simulink model "dt_toy_model_simulation"  (R2024a)
settings: Solver=FixedStepAuto  StartTime=0.0  StopTime=Tsim  FixedStep=dT  RelTol=1e-3
values from neighbouring files (symbols this model uses):
  Ac = full(sysA)    [CT_and_DT_Controller.m]
  Ad = dt_ol_sys.A    [CT_and_DT_Controller.m]
  Bc = full(sysB)    [CT_and_DT_Controller.m]
  Bd = dt_ol_sys.B    [CT_and_DT_Controller.m]
  dt_Phiu1 = full(dt_Phiu{1})    [CT_and_DT_Controller.m]
  dt_Phiu2 = full(dt_Phiu{2})    [CT_and_DT_Controller.m]
  dt_Phiu3 = full(dt_Phiu{3})    [CT_and_DT_Controller.m]
  dt_Phiu4 = full(dt_Phiu{4})    [CT_and_DT_Controller.m]
  dt_Phiu5 = full(dt_Phiu{5})    [CT_and_DT_Controller.m]
  dt_Phiu6 = full(dt_Phiu{6})    [CT_and_DT_Controller.m]
  dt_Phiu7 = full(dt_Phiu{7})    [CT_and_DT_Controller.m]
  dt_Phix2 = full(dt_Phix{2})    [CT_and_DT_Controller.m]
  dt_Phix3 = full(dt_Phix{3})    [CT_and_DT_Controller.m]
  dt_Phix4 = full(dt_Phix{4})    [CT_and_DT_Controller.m]
  dt_Phix5 = full(dt_Phix{5})    [CT_and_DT_Controller.m]
  dt_Phix6 = full(dt_Phix{6})    [CT_and_DT_Controller.m]
  dt_Phix7 = full(dt_Phix{7})    [CT_and_DT_Controller.m]
  Ts = 0.2    [CT_and_DT_Controller.m]
  x0 = zeros(n,1)    [CT_and_DT_Controller.m]
(part 1 of 2)
settings Model: Creator=ralph zhao  LastModifiedBy=ralph zhao

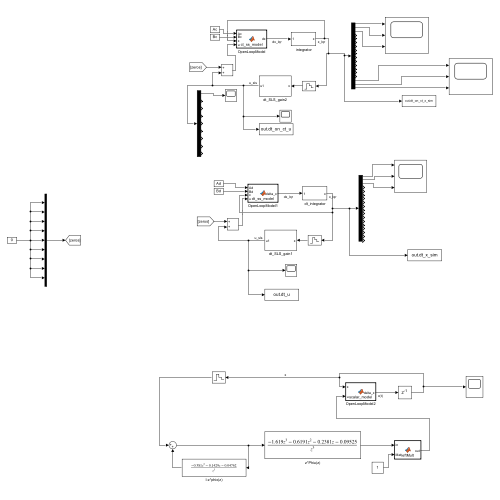
[thumbnail: Simulink's stored preview of the top-level diagram]
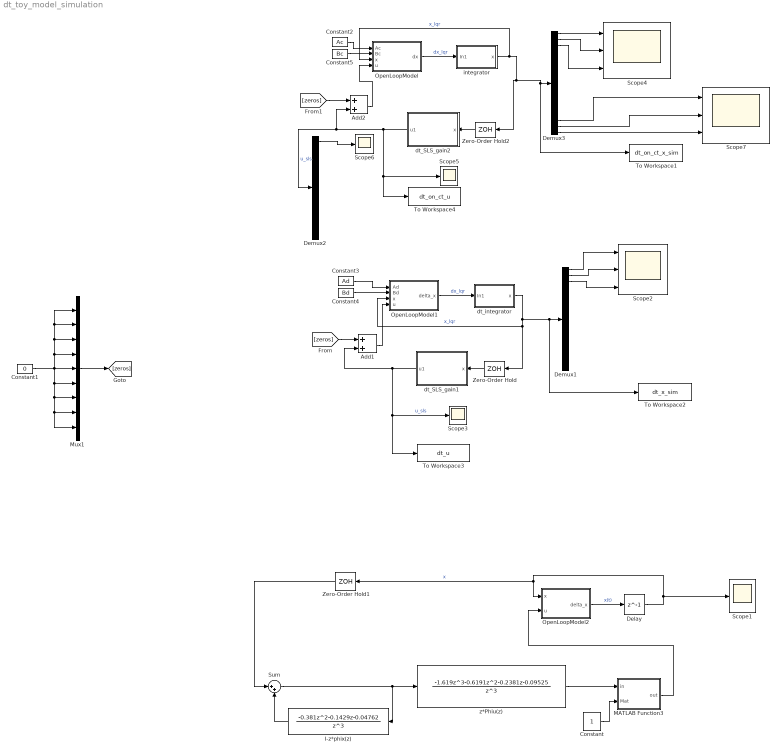
== system dt_toy_model_simulation ==
  " dt_integrator" : Subsystem
  " integrator" : Subsystem
  Add1 : Sum
  Add2 : Sum
  Constant : Constant
  Constant1 : Constant  Value=0
  Constant2 : Constant  Value=Ac
  Constant3 : Constant  Value=Ad
  Constant4 : Constant  Value=Bd
  Constant5 : Constant  Value=Bc
  Delay : Delay  DelayLength=1  InitialCondition=0.5
  Demux1 : Demux  Outputs=18
  Demux2 : Demux  Outputs=9
  Demux3 : Demux  Outputs=18
  I-z*phix(z) : DiscreteTransferFcn  Numerator=[-0.381 -0.1429 -0.04762]  Denominator=[1 0 0 0]
  MATLAB Function3 : MATLAB Function  TreatAsAtomicUnit=on
  Mux1 : Mux  Inputs=9
  OpenLoopModel : MATLAB Function  TreatAsAtomicUnit=on
  OpenLoopModel1 : MATLAB Function  TreatAsAtomicUnit=on
  OpenLoopModel2 : MATLAB Function  TreatAsAtomicUnit=on
  Scope{1,3,5..6} (4 alike) : Scope
  Scope2 : Scope  NumInputPorts=3
  Scope4 : Scope  NumInputPorts=3
  Scope7 : Scope  NumInputPorts=3
  Sum : Sum  Inputs=|++
  To Workspace1 : ToWorkspace  VariableName=dt_on_ct_x_sim  SaveFormat=Timeseries  SampleTime=-1
  To Workspace2 : ToWorkspace  VariableName=dt_x_sim  SaveFormat=Timeseries  SampleTime=-1
  To Workspace3 : ToWorkspace  VariableName=dt_u  SaveFormat=Timeseries  SampleTime=-1
  To Workspace4 : ToWorkspace  VariableName=dt_on_ct_u  SaveFormat=Timeseries  SampleTime=-1
  Zero-Order Hold : ZeroOrderHold  SampleTime=Ts
  Zero-Order Hold1 : ZeroOrderHold  SampleTime=Ts
  Zero-Order Hold2 : ZeroOrderHold  SampleTime=Ts
  dt_SLS_gain1 : Subsystem
  dt_SLS_gain2 : Subsystem
  z*Phiu(z) : DiscreteTransferFcn  Numerator=[-1.619 -0.6191 -0.2381 -0.09525]  Denominator=[1 0 0 0]
  wires:
  dt_SLS_gain1/1(u1) -> Add1/2, Scope3/1, To Workspace3/1  "u_sls"
  Add1/1 -> OpenLoopModel1/4(u)
  " dt_integrator"/1(x) -> OpenLoopModel1/3(x), Zero-Order Hold/1, Demux1/1, To Workspace2/1  "x_lqr"
  Mux1/1 -> [zeros]
  Demux1/3 -> Scope2/3
  Demux1/2 -> Scope2/2
  Demux1/1 -> Scope2/1
  OpenLoopModel1/1(delta_x) -> " dt_integrator"/1(In1)  "dx_lqr"
  Zero-Order Hold/1 -> dt_SLS_gain1/1(x)
  OpenLoopModel2/1(delta_x) -> Delay/1  "x(t)"
  Delay/1 -> Zero-Order Hold1/1, OpenLoopModel2/1(x), Scope1/1  "x"
  I-z*phix(z)/1 -> Sum/2
  Sum/1 -> I-z*phix(z)/1, z*Phiu(z)/1
  z*Phiu(z)/1 -> MATLAB Function3/1(in)
  Constant/1 -> MATLAB Function3/2(Mat)
  MATLAB Function3/1(out) -> OpenLoopModel2/2(u)
  Zero-Order Hold1/1 -> Sum/1
  Zero-Order Hold2/1 -> dt_SLS_gain2/1(x)
  OpenLoopModel/1(dx) -> " integrator"/1(In1)  "dx_lqr"
  " integrator"/1(x) -> OpenLoopModel/3(x), Zero-Order Hold2/1, To Workspace1/1, Demux3/1  "x_lqr"
  Add2/1 -> OpenLoopModel/4(u)
  dt_SLS_gain2/1(u1) -> To Workspace4/1, Scope5/1, Demux2/1, Add2/2  "u_sls"
  Constant3/1 -> OpenLoopModel1/1(Ad)
  Constant4/1 -> OpenLoopModel1/2(Bd)
  Constant1/1 -> Mux1/1, Mux1/2, Mux1/3, Mux1/4, Mux1/5, Mux1/6, Mux1/8, Mux1/9, Mux1/7
  [zeros] -> Add1/1
  [zeros] -> Add2/1
  Constant2/1 -> OpenLoopModel/1(Ac)
  Constant5/1 -> OpenLoopModel/2(Bc)
  Demux3/1 -> Scope4/1
  Demux3/2 -> Scope4/2
  Demux3/3 -> Scope4/3
  Demux2/1 -> Scope6/1
  Demux3/18 -> Scope7/3
  Demux3/17 -> Scope7/2
  Demux3/16 -> Scope7/1

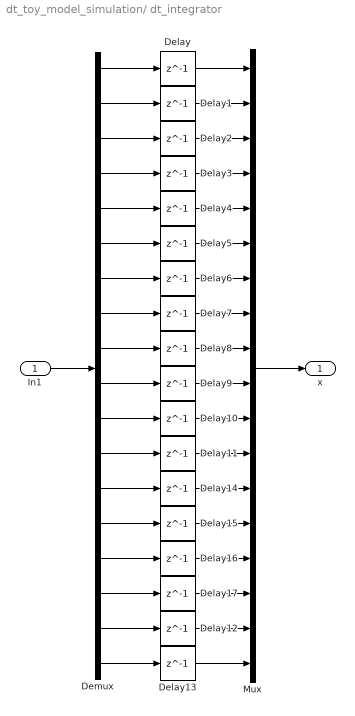
== system dt_toy_model_simulation/ dt_integrator ==
  In1 : Inport
  Delay : Delay  DelayLength=1  InitialCondition=x0(1)
  Delay1 : Delay  DelayLength=1  InitialCondition=x0(2)
  Delay10 : Delay  DelayLength=1  InitialCondition=x0(11)
  Delay11 : Delay  DelayLength=1  InitialCondition=x0(12)
  Delay12 : Delay  DelayLength=1  InitialCondition=x0(17)
  Delay13 : Delay  DelayLength=1  InitialCondition=x0(18)
  Delay14 : Delay  DelayLength=1  InitialCondition=x0(13)
  Delay15 : Delay  DelayLength=1  InitialCondition=x0(14)
  Delay16 : Delay  DelayLength=1  InitialCondition=x0(15)
  Delay17 : Delay  DelayLength=1  InitialCondition=x0(16)
  Delay2 : Delay  DelayLength=1  InitialCondition=x0(3)
  Delay3 : Delay  DelayLength=1  InitialCondition=x0(4)
  Delay4 : Delay  DelayLength=1  InitialCondition=x0(5)
  Delay5 : Delay  DelayLength=1  InitialCondition=x0(6)
  Delay6 : Delay  DelayLength=1  InitialCondition=x0(7)
  Delay7 : Delay  DelayLength=1  InitialCondition=x0(8)
  Delay8 : Delay  DelayLength=1  InitialCondition=x0(9)
  Delay9 : Delay  DelayLength=1  InitialCondition=x0(10)
  Demux : Demux  Outputs=18
  Mux : Mux  Inputs=18
  x : Outport
  wires:
  Delay2/1 -> Mux/3
  Delay1/1 -> Mux/2
  Delay/1 -> Mux/1
  Demux/3 -> Delay2/1
  In1/1 -> Demux/1
  Mux/1 -> x/1
  Demux/2 -> Delay1/1
  Demux/1 -> Delay/1
  Demux/18 -> Delay13/1
  Demux/4 -> Delay3/1
  Delay3/1 -> Mux/4
  Demux/5 -> Delay4/1
  Delay4/1 -> Mux/5
  Delay5/1 -> Mux/6
  Demux/6 -> Delay5/1
  Demux/7 -> Delay6/1
  Delay6/1 -> Mux/7
  Demux/14 -> Delay15/1
  Delay15/1 -> Mux/14
  Delay13/1 -> Mux/18
  Delay12/1 -> Mux/17
  Delay17/1 -> Mux/16
  Delay16/1 -> Mux/15
  Demux/15 -> Delay16/1
  Demux/16 -> Delay17/1
  Demux/17 -> Delay12/1
  Demux/8 -> Delay7/1
  Demux/9 -> Delay8/1
  Delay9/1 -> Mux/10
  Delay10/1 -> Mux/11
  Delay11/1 -> Mux/12
  Delay14/1 -> Mux/13
  Demux/13 -> Delay14/1
  Demux/12 -> Delay11/1
  Demux/11 -> Delay10/1
  Demux/10 -> Delay9/1
  Delay8/1 -> Mux/9
  Delay7/1 -> Mux/8

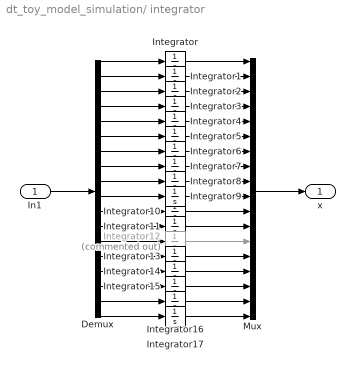
== system dt_toy_model_simulation/ integrator ==
  In1 : Inport
  Demux : Demux  Outputs=18
  Integrator : Integrator  InitialCondition=x0(1)
  Integrator1 : Integrator  InitialCondition=x0(2)
  Integrator10 : Integrator  InitialCondition=x0(11)
  Integrator11 : Integrator  InitialCondition=x0(12)
  Integrator12 : Integrator  Commented=on  InitialCondition=x0(13)
  Integrator13 : Integrator  InitialCondition=x0(14)
  Integrator14 : Integrator  InitialCondition=x0(15)
  Integrator15 : Integrator  InitialCondition=x0(16)
  Integrator16 : Integrator  InitialCondition=x0(17)
  Integrator17 : Integrator  InitialCondition=x0(18)
  Integrator2 : Integrator  InitialCondition=x0(3)
  Integrator3 : Integrator  InitialCondition=x0(4)
  Integrator4 : Integrator  InitialCondition=x0(5)
  Integrator5 : Integrator  InitialCondition=x0(6)
  Integrator6 : Integrator  InitialCondition=x0(7)
  Integrator7 : Integrator  InitialCondition=x0(8)
  Integrator8 : Integrator  InitialCondition=x0(9)
  Integrator9 : Integrator  InitialCondition=x0(10)
  Mux : Mux  Inputs=18
  x : Outport
  wires:
  Integrator2/1 -> Mux/3
  Integrator1/1 -> Mux/2
  Integrator/1 -> Mux/1
  Demux/3 -> Integrator2/1
  In1/1 -> Demux/1
  Mux/1 -> x/1
  Demux/2 -> Integrator1/1
  Demux/1 -> Integrator/1
  Demux/4 -> Integrator3/1
  Integrator3/1 -> Mux/4
  Demux/9 -> Integrator8/1
  Integrator8/1 -> Mux/9
  Demux/8 -> Integrator7/1
  Demux/7 -> Integrator6/1
  Demux/6 -> Integrator5/1
  Demux/5 -> Integrator4/1
  Integrator4/1 -> Mux/5
  Integrator5/1 -> Mux/6
  Integrator6/1 -> Mux/7
  Integrator7/1 -> Mux/8
  Demux/10 -> Integrator9/1
  Demux/11 -> Integrator10/1
  Demux/12 -> Integrator11/1
  Demux/13 -> Integrator12/1
  Demux/14 -> Integrator13/1
  Demux/15 -> Integrator14/1
  Demux/16 -> Integrator15/1
  Demux/17 -> Integrator16/1
  Demux/18 -> Integrator17/1
  Integrator17/1 -> Mux/18
  Integrator16/1 -> Mux/17
  Integrator15/1 -> Mux/16
  Integrator14/1 -> Mux/15
  Integrator13/1 -> Mux/14
  Integrator12/1 -> Mux/13
  Integrator11/1 -> Mux/12
  Integrator10/1 -> Mux/11
  Integrator9/1 -> Mux/10

== system dt_toy_model_simulation/dt_SLS_gain1 ==
  x : Inport
  Subtract1 : Sum  Inputs=+-
  z*Phi_u(z) : Subsystem
  z*Phi_x(z)-I : Subsystem
  u1 : Outport
  wires:
  z*Phi_u(z)/1(z*phi_u(z)) -> u1/1
  z*Phi_x(z)-I/1((z*phi_x(z)-I)) -> Subtract1/2
  Subtract1/1 -> z*Phi_x(z)-I/1(v), z*Phi_u(z)/1(I)  "v"
  x/1 -> Subtract1/1

== system dt_toy_model_simulation/dt_SLS_gain2 ==
  x : Inport
  Subtract1 : Sum  Inputs=+-
  z*Phi_u(z) : Subsystem
  z*Phi_x(z)-I : Subsystem
  u1 : Outport
  wires:
  x/1 -> Subtract1/1
  Subtract1/1 -> z*Phi_u(z)/1(I), z*Phi_x(z)-I/1(v)  "v"
  z*Phi_x(z)-I/1((z*phi_x(z)-I)) -> Subtract1/2
  z*Phi_u(z)/1(z*phi_u(z)) -> u1/1

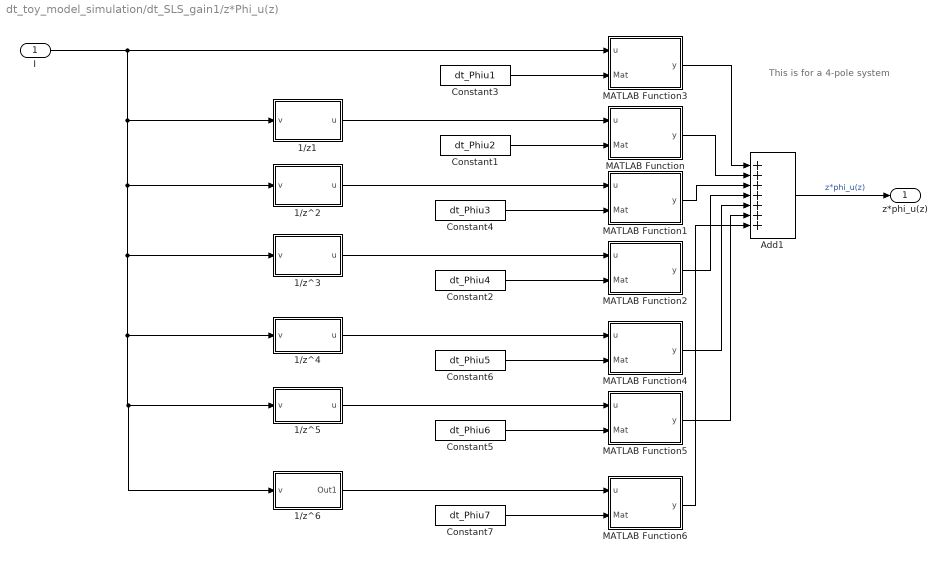
== system dt_toy_model_simulation/dt_SLS_gain1/z*Phi_u(z) ==
  note: This is for a 4-pole
      |  system
  I : Inport
  1/z1 : Subsystem
  1/z^2 : Subsystem
  1/z^3 : Subsystem
  1/z^4 : Subsystem
  1/z^5 : Subsystem
  1/z^6 : Subsystem
  Add1 : Sum  Inputs=+++++++
  Constant1 : Constant  Value=dt_Phiu2
  Constant2 : Constant  Value=dt_Phiu4
  Constant3 : Constant  Value=dt_Phiu1
  Constant4 : Constant  Value=dt_Phiu3
  Constant5 : Constant  Value=dt_Phiu6
  Constant6 : Constant  Value=dt_Phiu5
  Constant7 : Constant  Value=dt_Phiu7
  MATLAB Function : MATLAB Function  TreatAsAtomicUnit=on
  MATLAB Function1 : MATLAB Function  TreatAsAtomicUnit=on
  MATLAB Function2 : MATLAB Function  TreatAsAtomicUnit=on
  MATLAB Function3 : MATLAB Function  TreatAsAtomicUnit=on
  MATLAB Function4 : MATLAB Function  TreatAsAtomicUnit=on
  MATLAB Function5 : MATLAB Function  TreatAsAtomicUnit=on
  MATLAB Function6 : MATLAB Function  TreatAsAtomicUnit=on
  z*phi_u(z) : Outport
  wires:
  Constant7/1 -> MATLAB Function6/2(Mat)
  MATLAB Function6/1(y) -> Add1/7
  1/z^6/1(Out1) -> MATLAB Function6/1(u)
  I/1 -> MATLAB Function3/1(u), 1/z^2/1(v), 1/z^3/1(v), 1/z^5/1(v), 1/z^6/1(v), 1/z^4/1(v), 1/z1/1(v)
  Constant4/1 -> MATLAB Function1/2(Mat)
  1/z^2/1(u) -> MATLAB Function1/1(u)
  Constant1/1 -> MATLAB Function/2(Mat)
  Constant2/1 -> MATLAB Function2/2(Mat)
  1/z1/1(u) -> MATLAB Function/1(u)
  Add1/1 -> z*phi_u(z)/1  "z*phi_u(z)"
  MATLAB Function2/1(y) -> Add1/4
  MATLAB Function1/1(y) -> Add1/3
  MATLAB Function/1(y) -> Add1/2
  MATLAB Function3/1(y) -> Add1/1
  Constant3/1 -> MATLAB Function3/2(Mat)
  1/z^3/1(u) -> MATLAB Function2/1(u)
  1/z^5/1(u) -> MATLAB Function5/1(u)
  MATLAB Function4/1(y) -> Add1/5
  MATLAB Function5/1(y) -> Add1/6
  Constant5/1 -> MATLAB Function5/2(Mat)
  1/z^4/1(u) -> MATLAB Function4/1(u)
  Constant6/1 -> MATLAB Function4/2(Mat)

== system dt_toy_model_simulation/dt_SLS_gain1/z*Phi_x(z)-I ==
  note: This is for a 4-pole system
  v : Inport
  1/z : Subsystem
  1/z^2 : Subsystem
  1/z^3 : Subsystem
  1/z^4 : Subsystem
  1/z^5 : Subsystem
  1/z^6 : Subsystem
  Add1 : Sum  Inputs=++++++
  Constant1 : Constant  Value=dt_Phix2
  Constant2 : Constant  Value=dt_Phix4
  Constant3 : Constant  Value=dt_Phix7
  Constant4 : Constant  Value=dt_Phix3
  Constant5 : Constant  Value=dt_Phix6
  Constant6 : Constant  Value=dt_Phix5
  MATLAB Function : MATLAB Function  TreatAsAtomicUnit=on
  MATLAB Function1 : MATLAB Function  TreatAsAtomicUnit=on
  MATLAB Function2 : MATLAB Function  TreatAsAtomicUnit=on
  MATLAB Function3 : MATLAB Function  TreatAsAtomicUnit=on
  MATLAB Function4 : MATLAB Function  TreatAsAtomicUnit=on
  MATLAB Function5 : MATLAB Function  TreatAsAtomicUnit=on
  (z*phi_x(z)-I) : Outport
  wires:
  MATLAB Function3/1(y) -> Add1/6
  v/1 -> 1/z^5/1(v), 1/z^6/1(v), 1/z^4/1(v), 1/z^3/1(v), 1/z^2/1(v), 1/z/1(v)
  1/z^6/1(Out1) -> MATLAB Function3/1(u)
  Constant3/1 -> MATLAB Function3/2(Mat)
  1/z^2/1(Out1) -> MATLAB Function1/1(u)
  Add1/1 -> (z*phi_x(z)-I)/1
  Constant1/1 -> MATLAB Function/2(Mat)
  1/z/1(Out1) -> MATLAB Function/1(u)
  MATLAB Function/1(y) -> Add1/1
  Constant4/1 -> MATLAB Function1/2(Mat)
  MATLAB Function1/1(y) -> Add1/2
  1/z^3/1(Out1) -> MATLAB Function2/1(u)
  Constant2/1 -> MATLAB Function2/2(Mat)
  MATLAB Function2/1(y) -> Add1/3
  Constant5/1 -> MATLAB Function5/2(Mat)
  1/z^5/1(Out1) -> MATLAB Function5/1(u)
  Constant6/1 -> MATLAB Function4/2(Mat)
  1/z^4/1(Out1) -> MATLAB Function4/1(u)
  MATLAB Function4/1(y) -> Add1/4
  MATLAB Function5/1(y) -> Add1/5

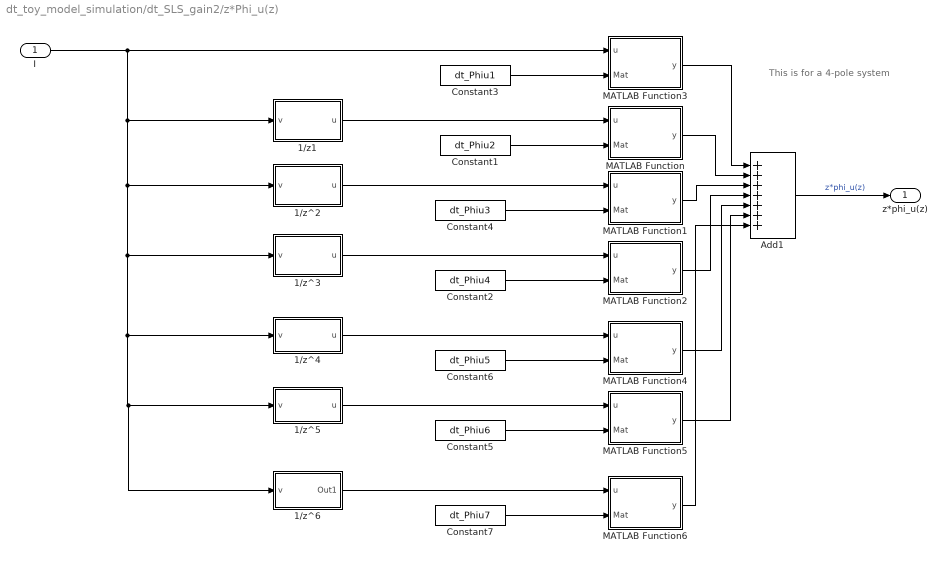
== system dt_toy_model_simulation/dt_SLS_gain2/z*Phi_u(z) ==
  note: This is for a 4-pole
      |  system
  I : Inport
  1/z1 : Subsystem
  1/z^2 : Subsystem
  1/z^3 : Subsystem
  1/z^4 : Subsystem
  1/z^5 : Subsystem
  1/z^6 : Subsystem
  Add1 : Sum  Inputs=+++++++
  Constant1 : Constant  Value=dt_Phiu2
  Constant2 : Constant  Value=dt_Phiu4
  Constant3 : Constant  Value=dt_Phiu1
  Constant4 : Constant  Value=dt_Phiu3
  Constant5 : Constant  Value=dt_Phiu6
  Constant6 : Constant  Value=dt_Phiu5
  Constant7 : Constant  Value=dt_Phiu7
  MATLAB Function : MATLAB Function  TreatAsAtomicUnit=on
  MATLAB Function1 : MATLAB Function  TreatAsAtomicUnit=on
  MATLAB Function2 : MATLAB Function  TreatAsAtomicUnit=on
  MATLAB Function3 : MATLAB Function  TreatAsAtomicUnit=on
  MATLAB Function4 : MATLAB Function  TreatAsAtomicUnit=on
  MATLAB Function5 : MATLAB Function  TreatAsAtomicUnit=on
  MATLAB Function6 : MATLAB Function  TreatAsAtomicUnit=on
  z*phi_u(z) : Outport
  wires:
  Constant6/1 -> MATLAB Function4/2(Mat)
  1/z^4/1(u) -> MATLAB Function4/1(u)
  Constant5/1 -> MATLAB Function5/2(Mat)
  MATLAB Function5/1(y) -> Add1/6
  MATLAB Function4/1(y) -> Add1/5
  1/z^5/1(u) -> MATLAB Function5/1(u)
  1/z^3/1(u) -> MATLAB Function2/1(u)
  Constant3/1 -> MATLAB Function3/2(Mat)
  MATLAB Function3/1(y) -> Add1/1
  MATLAB Function/1(y) -> Add1/2
  MATLAB Function1/1(y) -> Add1/3
  MATLAB Function2/1(y) -> Add1/4
  Add1/1 -> z*phi_u(z)/1  "z*phi_u(z)"
  1/z1/1(u) -> MATLAB Function/1(u)
  Constant2/1 -> MATLAB Function2/2(Mat)
  Constant1/1 -> MATLAB Function/2(Mat)
  1/z^2/1(u) -> MATLAB Function1/1(u)
  Constant4/1 -> MATLAB Function1/2(Mat)
  I/1 -> 1/z1/1(v), 1/z^4/1(v), 1/z^6/1(v), 1/z^5/1(v), 1/z^3/1(v), 1/z^2/1(v), MATLAB Function3/1(u)
  1/z^6/1(Out1) -> MATLAB Function6/1(u)
  MATLAB Function6/1(y) -> Add1/7
  Constant7/1 -> MATLAB Function6/2(Mat)

== system dt_toy_model_simulation/dt_SLS_gain2/z*Phi_x(z)-I ==
  note: This is for a 4-pole system
  v : Inport
  1/z : Subsystem
  1/z^2 : Subsystem
  1/z^3 : Subsystem
  1/z^4 : Subsystem
  1/z^5 : Subsystem
  1/z^6 : Subsystem
  Add1 : Sum  Inputs=++++++
  Constant1 : Constant  Value=dt_Phix2
  Constant2 : Constant  Value=dt_Phix4
  Constant3 : Constant  Value=dt_Phix7
  Constant4 : Constant  Value=dt_Phix3
  Constant5 : Constant  Value=dt_Phix6
  Constant6 : Constant  Value=dt_Phix5
  MATLAB Function : MATLAB Function  TreatAsAtomicUnit=on
  MATLAB Function1 : MATLAB Function  TreatAsAtomicUnit=on
  MATLAB Function2 : MATLAB Function  TreatAsAtomicUnit=on
  MATLAB Function3 : MATLAB Function  TreatAsAtomicUnit=on
  MATLAB Function4 : MATLAB Function  TreatAsAtomicUnit=on
  MATLAB Function5 : MATLAB Function  TreatAsAtomicUnit=on
  (z*phi_x(z)-I) : Outport
  wires:
  MATLAB Function5/1(y) -> Add1/5
  MATLAB Function4/1(y) -> Add1/4
  1/z^4/1(Out1) -> MATLAB Function4/1(u)
  Constant6/1 -> MATLAB Function4/2(Mat)
  1/z^5/1(Out1) -> MATLAB Function5/1(u)
  Constant5/1 -> MATLAB Function5/2(Mat)
  MATLAB Function2/1(y) -> Add1/3
  Constant2/1 -> MATLAB Function2/2(Mat)
  1/z^3/1(Out1) -> MATLAB Function2/1(u)
  MATLAB Function1/1(y) -> Add1/2
  Constant4/1 -> MATLAB Function1/2(Mat)
  MATLAB Function/1(y) -> Add1/1
  1/z/1(Out1) -> MATLAB Function/1(u)
  Constant1/1 -> MATLAB Function/2(Mat)
  Add1/1 -> (z*phi_x(z)-I)/1
  1/z^2/1(Out1) -> MATLAB Function1/1(u)
  Constant3/1 -> MATLAB Function3/2(Mat)
  1/z^6/1(Out1) -> MATLAB Function3/1(u)
  v/1 -> 1/z/1(v), 1/z^2/1(v), 1/z^3/1(v), 1/z^4/1(v), 1/z^6/1(v), 1/z^5/1(v)
  MATLAB Function3/1(y) -> Add1/6

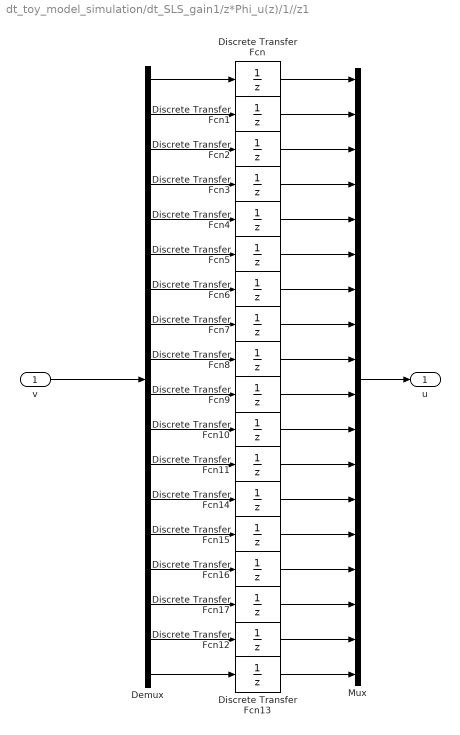
== system dt_toy_model_simulation/dt_SLS_gain1/z*Phi_u(z)/1//z1 ==
  v : Inport
  Demux : Demux  Outputs=18
  Discrete Transfer Fcn{,1..17} (18 alike) : DiscreteTransferFcn  Denominator=[1 0]
  Mux : Mux  Inputs=18
  u : Outport
  wires:
  Discrete Transfer Fcn1/1 -> Mux/2
  Demux/1 -> Discrete Transfer Fcn/1
  Discrete Transfer Fcn2/1 -> Mux/3
  Discrete Transfer Fcn/1 -> Mux/1
  Demux/2 -> Discrete Transfer Fcn1/1
  Demux/3 -> Discrete Transfer Fcn2/1
  Mux/1 -> u/1
  v/1 -> Demux/1
  Demux/4 -> Discrete Transfer Fcn3/1
  Demux/5 -> Discrete Transfer Fcn4/1
  Demux/6 -> Discrete Transfer Fcn5/1
  Demux/7 -> Discrete Transfer Fcn6/1
  Demux/8 -> Discrete Transfer Fcn7/1
  Demux/9 -> Discrete Transfer Fcn8/1
  Demux/10 -> Discrete Transfer Fcn9/1
  Demux/11 -> Discrete Transfer Fcn10/1
  Demux/12 -> Discrete Transfer Fcn11/1
  Demux/13 -> Discrete Transfer Fcn14/1
  Demux/14 -> Discrete Transfer Fcn15/1
  Demux/15 -> Discrete Transfer Fcn16/1
  Demux/16 -> Discrete Transfer Fcn17/1
  Demux/17 -> Discrete Transfer Fcn12/1
  Demux/18 -> Discrete Transfer Fcn13/1
  Discrete Transfer Fcn13/1 -> Mux/18
  Discrete Transfer Fcn12/1 -> Mux/17
  Discrete Transfer Fcn17/1 -> Mux/16
  Discrete Transfer Fcn16/1 -> Mux/15
  Discrete Transfer Fcn15/1 -> Mux/14
  Discrete Transfer Fcn14/1 -> Mux/13
  Discrete Transfer Fcn3/1 -> Mux/4
  Discrete Transfer Fcn4/1 -> Mux/5
  Discrete Transfer Fcn5/1 -> Mux/6
  Discrete Transfer Fcn6/1 -> Mux/7
  Discrete Transfer Fcn7/1 -> Mux/8
  Discrete Transfer Fcn8/1 -> Mux/9
  Discrete Transfer Fcn9/1 -> Mux/10
  Discrete Transfer Fcn10/1 -> Mux/11
  Discrete Transfer Fcn11/1 -> Mux/12

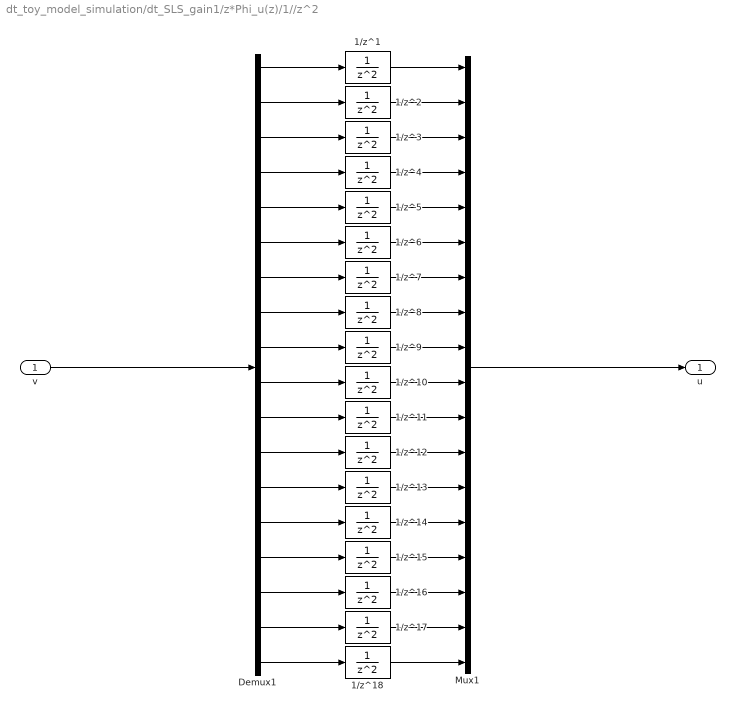
== system dt_toy_model_simulation/dt_SLS_gain1/z*Phi_u(z)/1//z^2 ==
  v : Inport
  1/z^{1..18} (18 alike) : DiscreteTransferFcn  Denominator=[1 0 0]
  Demux1 : Demux  Outputs=18
  Mux1 : Mux  Inputs=18
  u : Outport
  wires:
  Demux1/7 -> 1/z^7/1
  1/z^16/1 -> Mux1/16
  Demux1/10 -> 1/z^10/1
  1/z^17/1 -> Mux1/17
  Demux1/14 -> 1/z^14/1
  Demux1/6 -> 1/z^6/1
  1/z^13/1 -> Mux1/13
  Mux1/1 -> u/1
  Demux1/2 -> 1/z^2/1
  Demux1/1 -> 1/z^1/1
  1/z^1/1 -> Mux1/1
  1/z^6/1 -> Mux1/6
  Demux1/13 -> 1/z^13/1
  1/z^11/1 -> Mux1/11
  1/z^15/1 -> Mux1/15
  1/z^7/1 -> Mux1/7
  Demux1/12 -> 1/z^12/1
  1/z^5/1 -> Mux1/5
  Demux1/5 -> 1/z^5/1
  Demux1/9 -> 1/z^9/1
  1/z^10/1 -> Mux1/10
  Demux1/16 -> 1/z^16/1
  Demux1/4 -> 1/z^4/1
  1/z^14/1 -> Mux1/14
  1/z^2/1 -> Mux1/2
  1/z^18/1 -> Mux1/18
  v/1 -> Demux1/1
  Demux1/8 -> 1/z^8/1
  1/z^3/1 -> Mux1/3
  1/z^12/1 -> Mux1/12
  1/z^8/1 -> Mux1/8
  1/z^4/1 -> Mux1/4
  Demux1/3 -> 1/z^3/1
  Demux1/11 -> 1/z^11/1
  Demux1/18 -> 1/z^18/1
  1/z^9/1 -> Mux1/9
  Demux1/17 -> 1/z^17/1
  Demux1/15 -> 1/z^15/1

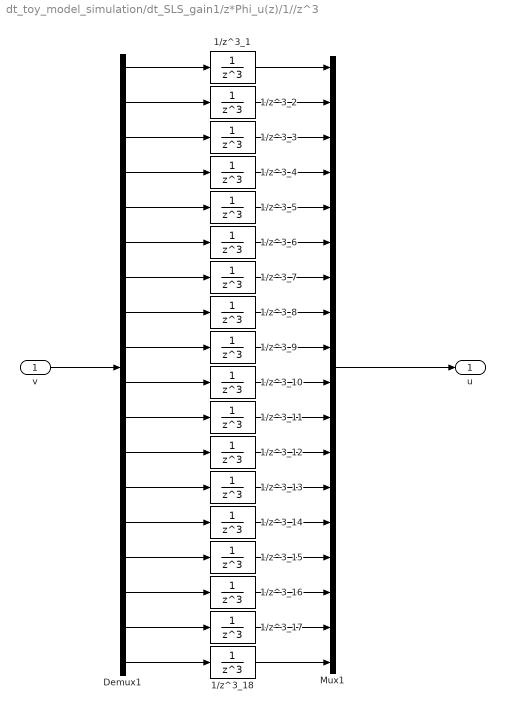
== system dt_toy_model_simulation/dt_SLS_gain1/z*Phi_u(z)/1//z^3 ==
  v : Inport
  1/z^3_{1..18} (18 alike) : DiscreteTransferFcn  Denominator=[1 0 0 0]
  Demux1 : Demux  Outputs=18
  Mux1 : Mux  Inputs=18
  u : Outport
  wires:
  Demux1/8 -> 1/z^3_8/1
  1/z^3_8/1 -> Mux1/8
  Demux1/4 -> 1/z^3_4/1
  1/z^3_5/1 -> Mux1/5
  1/z^3_18/1 -> Mux1/18
  1/z^3_17/1 -> Mux1/17
  Demux1/5 -> 1/z^3_5/1
  Demux1/17 -> 1/z^3_17/1
  Demux1/14 -> 1/z^3_14/1
  1/z^3_16/1 -> Mux1/16
  1/z^3_14/1 -> Mux1/14
  Demux1/11 -> 1/z^3_11/1
  1/z^3_11/1 -> Mux1/11
  Demux1/16 -> 1/z^3_16/1
  1/z^3_4/1 -> Mux1/4
  1/z^3_10/1 -> Mux1/10
  Demux1/18 -> 1/z^3_18/1
  Demux1/13 -> 1/z^3_13/1
  1/z^3_13/1 -> Mux1/13
  1/z^3_12/1 -> Mux1/12
  Demux1/12 -> 1/z^3_12/1
  Demux1/15 -> 1/z^3_15/1
  1/z^3_15/1 -> Mux1/15
  Mux1/1 -> u/1
  1/z^3_6/1 -> Mux1/6
  1/z^3_2/1 -> Mux1/2
  Demux1/2 -> 1/z^3_2/1
  Demux1/6 -> 1/z^3_6/1
  v/1 -> Demux1/1
  1/z^3_1/1 -> Mux1/1
  Demux1/10 -> 1/z^3_10/1
  Demux1/1 -> 1/z^3_1/1
  1/z^3_3/1 -> Mux1/3
  1/z^3_7/1 -> Mux1/7
  Demux1/7 -> 1/z^3_7/1
  Demux1/9 -> 1/z^3_9/1
  1/z^3_9/1 -> Mux1/9
  Demux1/3 -> 1/z^3_3/1

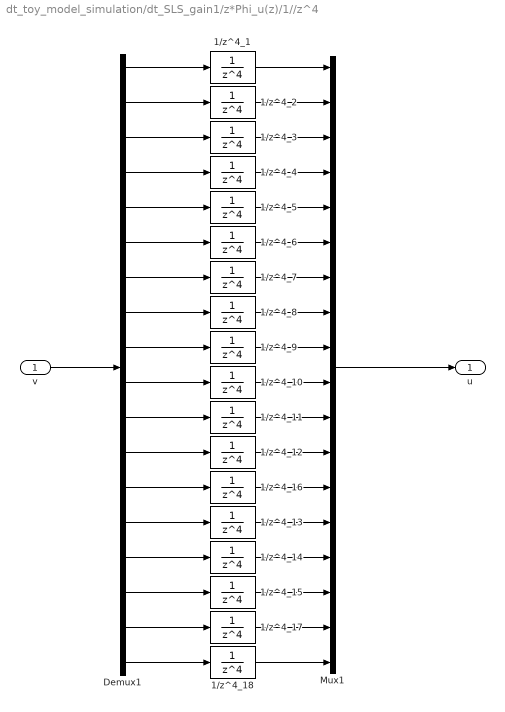
== system dt_toy_model_simulation/dt_SLS_gain1/z*Phi_u(z)/1//z^4 ==
  v : Inport
  1/z^4_{1..18} (18 alike) : DiscreteTransferFcn  Denominator=[1 0 0 0 0]
  Demux1 : Demux  Outputs=18
  Mux1 : Mux  Inputs=18
  u : Outport
  wires:
  Demux1/3 -> 1/z^4_3/1
  1/z^4_9/1 -> Mux1/9
  Demux1/9 -> 1/z^4_9/1
  Demux1/7 -> 1/z^4_7/1
  1/z^4_7/1 -> Mux1/7
  1/z^4_3/1 -> Mux1/3
  Demux1/1 -> 1/z^4_1/1
  Demux1/10 -> 1/z^4_10/1
  1/z^4_1/1 -> Mux1/1
  v/1 -> Demux1/1
  Demux1/6 -> 1/z^4_6/1
  Demux1/2 -> 1/z^4_2/1
  1/z^4_2/1 -> Mux1/2
  1/z^4_6/1 -> Mux1/6
  Mux1/1 -> u/1
  1/z^4_14/1 -> Mux1/15
  Demux1/15 -> 1/z^4_14/1
  Demux1/12 -> 1/z^4_12/1
  1/z^4_12/1 -> Mux1/12
  1/z^4_16/1 -> Mux1/13
  Demux1/13 -> 1/z^4_16/1
  Demux1/18 -> 1/z^4_18/1
  1/z^4_10/1 -> Mux1/10
  1/z^4_4/1 -> Mux1/4
  Demux1/16 -> 1/z^4_15/1
  1/z^4_11/1 -> Mux1/11
  Demux1/11 -> 1/z^4_11/1
  1/z^4_13/1 -> Mux1/14
  1/z^4_15/1 -> Mux1/16
  Demux1/14 -> 1/z^4_13/1
  Demux1/17 -> 1/z^4_17/1
  Demux1/5 -> 1/z^4_5/1
  1/z^4_17/1 -> Mux1/17
  1/z^4_18/1 -> Mux1/18
  1/z^4_5/1 -> Mux1/5
  Demux1/4 -> 1/z^4_4/1
  1/z^4_8/1 -> Mux1/8
  Demux1/8 -> 1/z^4_8/1

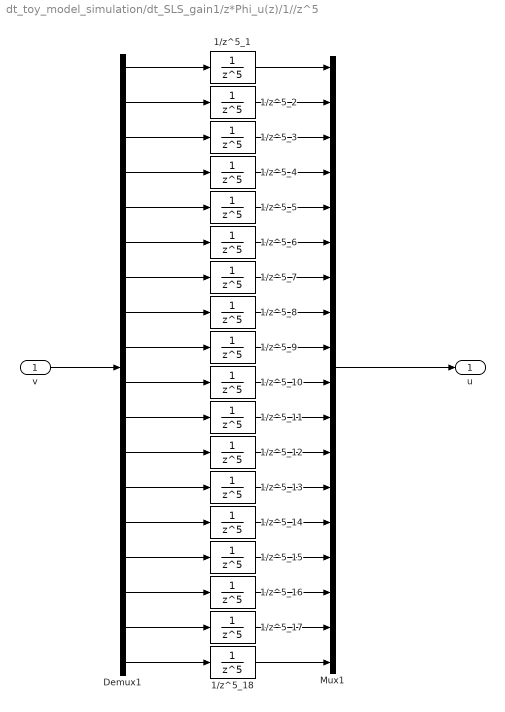
== system dt_toy_model_simulation/dt_SLS_gain1/z*Phi_u(z)/1//z^5 ==
  v : Inport
  1/z^5_{1..18} (18 alike) : DiscreteTransferFcn  Denominator=[1 0 0 0 0 0]
  Demux1 : Demux  Outputs=18
  Mux1 : Mux  Inputs=18
  u : Outport
  wires:
  Demux1/8 -> 1/z^5_8/1
  1/z^5_8/1 -> Mux1/8
  Demux1/4 -> 1/z^5_4/1
  1/z^5_5/1 -> Mux1/5
  1/z^5_18/1 -> Mux1/18
  1/z^5_17/1 -> Mux1/17
  Demux1/5 -> 1/z^5_5/1
  Demux1/17 -> 1/z^5_17/1
  Demux1/14 -> 1/z^5_14/1
  1/z^5_16/1 -> Mux1/16
  1/z^5_14/1 -> Mux1/14
  Demux1/11 -> 1/z^5_11/1
  1/z^5_11/1 -> Mux1/11
  Demux1/16 -> 1/z^5_16/1
  1/z^5_4/1 -> Mux1/4
  1/z^5_10/1 -> Mux1/10
  Demux1/18 -> 1/z^5_18/1
  Demux1/13 -> 1/z^5_13/1
  1/z^5_13/1 -> Mux1/13
  1/z^5_12/1 -> Mux1/12
  Demux1/12 -> 1/z^5_12/1
  Demux1/15 -> 1/z^5_15/1
  1/z^5_15/1 -> Mux1/15
  Mux1/1 -> u/1
  1/z^5_6/1 -> Mux1/6
  1/z^5_2/1 -> Mux1/2
  Demux1/2 -> 1/z^5_2/1
  Demux1/6 -> 1/z^5_6/1
  v/1 -> Demux1/1
  1/z^5_1/1 -> Mux1/1
  Demux1/10 -> 1/z^5_10/1
  Demux1/1 -> 1/z^5_1/1
  1/z^5_3/1 -> Mux1/3
  1/z^5_7/1 -> Mux1/7
  Demux1/7 -> 1/z^5_7/1
  Demux1/9 -> 1/z^5_9/1
  1/z^5_9/1 -> Mux1/9
  Demux1/3 -> 1/z^5_3/1

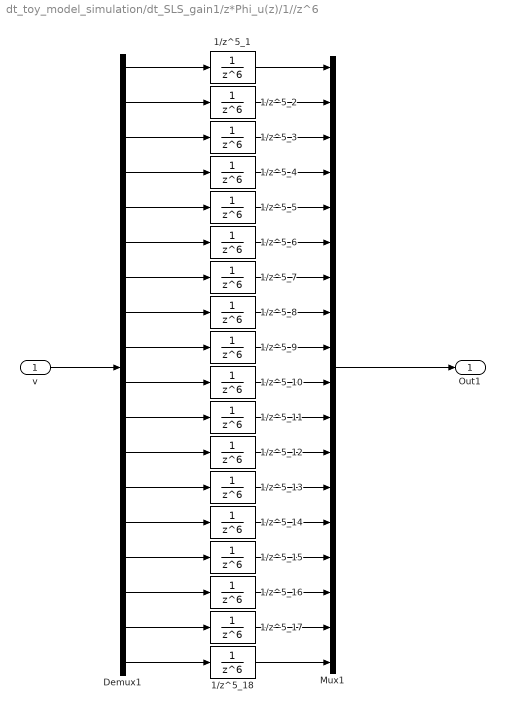
== system dt_toy_model_simulation/dt_SLS_gain1/z*Phi_u(z)/1//z^6 ==
  v : Inport
  1/z^5_{1..18} (18 alike) : DiscreteTransferFcn  Denominator=[1 0 0 0 0 0 0]
  Demux1 : Demux  Outputs=18
  Mux1 : Mux  Inputs=18
  Out1 : Outport
  wires:
  Demux1/3 -> 1/z^5_3/1
  1/z^5_9/1 -> Mux1/9
  Demux1/9 -> 1/z^5_9/1
  Demux1/7 -> 1/z^5_7/1
  1/z^5_7/1 -> Mux1/7
  1/z^5_3/1 -> Mux1/3
  Demux1/1 -> 1/z^5_1/1
  Demux1/10 -> 1/z^5_10/1
  1/z^5_1/1 -> Mux1/1
  v/1 -> Demux1/1
  Demux1/6 -> 1/z^5_6/1
  Demux1/2 -> 1/z^5_2/1
  1/z^5_2/1 -> Mux1/2
  1/z^5_6/1 -> Mux1/6
  Mux1/1 -> Out1/1
  1/z^5_15/1 -> Mux1/15
  Demux1/15 -> 1/z^5_15/1
  Demux1/12 -> 1/z^5_12/1
  1/z^5_12/1 -> Mux1/12
  1/z^5_13/1 -> Mux1/13
  Demux1/13 -> 1/z^5_13/1
  Demux1/18 -> 1/z^5_18/1
  1/z^5_10/1 -> Mux1/10
  1/z^5_4/1 -> Mux1/4
  Demux1/16 -> 1/z^5_16/1
  1/z^5_11/1 -> Mux1/11
  Demux1/11 -> 1/z^5_11/1
  1/z^5_14/1 -> Mux1/14
  1/z^5_16/1 -> Mux1/16
  Demux1/14 -> 1/z^5_14/1
  Demux1/17 -> 1/z^5_17/1
  Demux1/5 -> 1/z^5_5/1
  1/z^5_17/1 -> Mux1/17
  1/z^5_18/1 -> Mux1/18
  1/z^5_5/1 -> Mux1/5
  Demux1/4 -> 1/z^5_4/1
  1/z^5_8/1 -> Mux1/8
  Demux1/8 -> 1/z^5_8/1

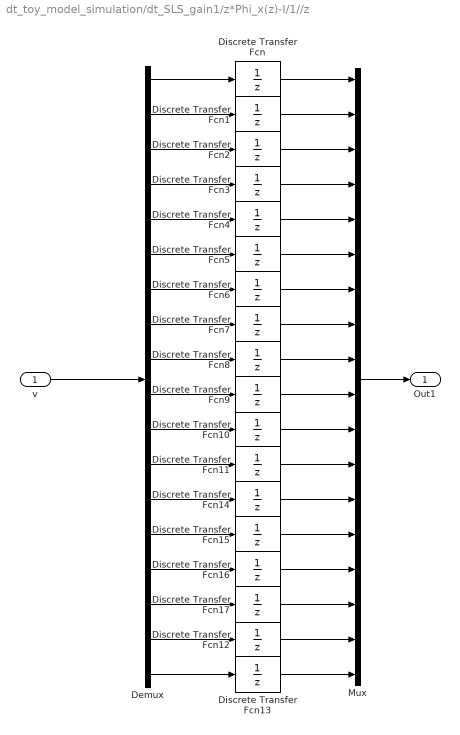
== system dt_toy_model_simulation/dt_SLS_gain1/z*Phi_x(z)-I/1//z ==
  v : Inport
  Demux : Demux  Outputs=18
  Discrete Transfer Fcn{,1..17} (18 alike) : DiscreteTransferFcn  Denominator=[1 0]
  Mux : Mux  Inputs=18
  Out1 : Outport
  wires:
  Discrete Transfer Fcn1/1 -> Mux/2
  Demux/1 -> Discrete Transfer Fcn/1
  Discrete Transfer Fcn2/1 -> Mux/3
  Discrete Transfer Fcn/1 -> Mux/1
  Demux/2 -> Discrete Transfer Fcn1/1
  Demux/3 -> Discrete Transfer Fcn2/1
  Mux/1 -> Out1/1
  v/1 -> Demux/1
  Demux/4 -> Discrete Transfer Fcn3/1
  Demux/5 -> Discrete Transfer Fcn4/1
  Demux/6 -> Discrete Transfer Fcn5/1
  Demux/7 -> Discrete Transfer Fcn6/1
  Demux/8 -> Discrete Transfer Fcn7/1
  Demux/9 -> Discrete Transfer Fcn8/1
  Demux/10 -> Discrete Transfer Fcn9/1
  Demux/11 -> Discrete Transfer Fcn10/1
  Demux/12 -> Discrete Transfer Fcn11/1
  Demux/13 -> Discrete Transfer Fcn14/1
  Demux/14 -> Discrete Transfer Fcn15/1
  Demux/15 -> Discrete Transfer Fcn16/1
  Demux/16 -> Discrete Transfer Fcn17/1
  Demux/17 -> Discrete Transfer Fcn12/1
  Demux/18 -> Discrete Transfer Fcn13/1
  Discrete Transfer Fcn13/1 -> Mux/18
  Discrete Transfer Fcn12/1 -> Mux/17
  Discrete Transfer Fcn17/1 -> Mux/16
  Discrete Transfer Fcn16/1 -> Mux/15
  Discrete Transfer Fcn15/1 -> Mux/14
  Discrete Transfer Fcn14/1 -> Mux/13
  Discrete Transfer Fcn3/1 -> Mux/4
  Discrete Transfer Fcn4/1 -> Mux/5
  Discrete Transfer Fcn5/1 -> Mux/6
  Discrete Transfer Fcn6/1 -> Mux/7
  Discrete Transfer Fcn7/1 -> Mux/8
  Discrete Transfer Fcn8/1 -> Mux/9
  Discrete Transfer Fcn9/1 -> Mux/10
  Discrete Transfer Fcn10/1 -> Mux/11
  Discrete Transfer Fcn11/1 -> Mux/12

== system dt_toy_model_simulation/dt_SLS_gain1/z*Phi_x(z)-I/1//z^2 ==
  v : Inport
  1/z^{1..18} (18 alike) : DiscreteTransferFcn  Denominator=[1 0 0]
  Demux1 : Demux  Outputs=18
  Mux1 : Mux  Inputs=18
  Out1 : Outport
  wires:
  Demux1/7 -> 1/z^7/1
  1/z^16/1 -> Mux1/16
  Demux1/10 -> 1/z^10/1
  1/z^17/1 -> Mux1/17
  Demux1/14 -> 1/z^14/1
  Demux1/6 -> 1/z^6/1
  1/z^13/1 -> Mux1/13
  Mux1/1 -> Out1/1
  Demux1/2 -> 1/z^2/1
  Demux1/1 -> 1/z^1/1
  1/z^1/1 -> Mux1/1
  1/z^6/1 -> Mux1/6
  Demux1/13 -> 1/z^13/1
  1/z^11/1 -> Mux1/11
  1/z^15/1 -> Mux1/15
  1/z^7/1 -> Mux1/7
  Demux1/12 -> 1/z^12/1
  1/z^5/1 -> Mux1/5
  Demux1/5 -> 1/z^5/1
  Demux1/9 -> 1/z^9/1
  1/z^10/1 -> Mux1/10
  Demux1/16 -> 1/z^16/1
  Demux1/4 -> 1/z^4/1
  1/z^14/1 -> Mux1/14
  1/z^2/1 -> Mux1/2
  1/z^18/1 -> Mux1/18
  v/1 -> Demux1/1
  Demux1/8 -> 1/z^8/1
  1/z^3/1 -> Mux1/3
  1/z^12/1 -> Mux1/12
  1/z^8/1 -> Mux1/8
  1/z^4/1 -> Mux1/4
  Demux1/3 -> 1/z^3/1
  Demux1/11 -> 1/z^11/1
  Demux1/18 -> 1/z^18/1
  1/z^9/1 -> Mux1/9
  Demux1/17 -> 1/z^17/1
  Demux1/15 -> 1/z^15/1

== system dt_toy_model_simulation/dt_SLS_gain1/z*Phi_x(z)-I/1//z^3 ==
  v : Inport
  1/z^3_{1..18} (18 alike) : DiscreteTransferFcn  Denominator=[1 0 0 0]
  Demux1 : Demux  Outputs=18
  Mux1 : Mux  Inputs=18
  Out1 : Outport
  wires:
  Demux1/8 -> 1/z^3_8/1
  1/z^3_8/1 -> Mux1/8
  Demux1/4 -> 1/z^3_4/1
  1/z^3_5/1 -> Mux1/5
  1/z^3_18/1 -> Mux1/18
  1/z^3_17/1 -> Mux1/17
  Demux1/5 -> 1/z^3_5/1
  Demux1/17 -> 1/z^3_17/1
  Demux1/14 -> 1/z^3_14/1
  1/z^3_16/1 -> Mux1/16
  1/z^3_14/1 -> Mux1/14
  Demux1/11 -> 1/z^3_11/1
  1/z^3_11/1 -> Mux1/11
  Demux1/16 -> 1/z^3_16/1
  1/z^3_4/1 -> Mux1/4
  1/z^3_10/1 -> Mux1/10
  Demux1/18 -> 1/z^3_18/1
  Demux1/13 -> 1/z^3_13/1
  1/z^3_13/1 -> Mux1/13
  1/z^3_12/1 -> Mux1/12
  Demux1/12 -> 1/z^3_12/1
  Demux1/15 -> 1/z^3_15/1
  1/z^3_15/1 -> Mux1/15
  Mux1/1 -> Out1/1
  1/z^3_6/1 -> Mux1/6
  1/z^3_2/1 -> Mux1/2
  Demux1/2 -> 1/z^3_2/1
  Demux1/6 -> 1/z^3_6/1
  v/1 -> Demux1/1
  1/z^3_1/1 -> Mux1/1
  Demux1/10 -> 1/z^3_10/1
  Demux1/1 -> 1/z^3_1/1
  1/z^3_3/1 -> Mux1/3
  1/z^3_7/1 -> Mux1/7
  Demux1/7 -> 1/z^3_7/1
  Demux1/9 -> 1/z^3_9/1
  1/z^3_9/1 -> Mux1/9
  Demux1/3 -> 1/z^3_3/1

== system dt_toy_model_simulation/dt_SLS_gain1/z*Phi_x(z)-I/1//z^4 ==
  v : Inport
  1/z^4_{1..18} (18 alike) : DiscreteTransferFcn  Denominator=[1 0 0 0 0]
  Demux1 : Demux  Outputs=18
  Mux1 : Mux  Inputs=18
  Out1 : Outport
  wires:
  Demux1/3 -> 1/z^4_3/1
  1/z^4_9/1 -> Mux1/9
  Demux1/9 -> 1/z^4_9/1
  Demux1/7 -> 1/z^4_7/1
  1/z^4_7/1 -> Mux1/7
  1/z^4_3/1 -> Mux1/3
  Demux1/1 -> 1/z^4_1/1
  Demux1/10 -> 1/z^4_10/1
  1/z^4_1/1 -> Mux1/1
  v/1 -> Demux1/1
  Demux1/6 -> 1/z^4_6/1
  Demux1/2 -> 1/z^4_2/1
  1/z^4_2/1 -> Mux1/2
  1/z^4_6/1 -> Mux1/6
  Mux1/1 -> Out1/1
  1/z^4_14/1 -> Mux1/15
  Demux1/15 -> 1/z^4_14/1
  Demux1/12 -> 1/z^4_12/1
  1/z^4_12/1 -> Mux1/12
  1/z^4_16/1 -> Mux1/13
  Demux1/13 -> 1/z^4_16/1
  Demux1/18 -> 1/z^4_18/1
  1/z^4_10/1 -> Mux1/10
  1/z^4_4/1 -> Mux1/4
  Demux1/16 -> 1/z^4_15/1
  1/z^4_11/1 -> Mux1/11
  Demux1/11 -> 1/z^4_11/1
  1/z^4_13/1 -> Mux1/14
  1/z^4_15/1 -> Mux1/16
  Demux1/14 -> 1/z^4_13/1
  Demux1/17 -> 1/z^4_17/1
  Demux1/5 -> 1/z^4_5/1
  1/z^4_17/1 -> Mux1/17
  1/z^4_18/1 -> Mux1/18
  1/z^4_5/1 -> Mux1/5
  Demux1/4 -> 1/z^4_4/1
  1/z^4_8/1 -> Mux1/8
  Demux1/8 -> 1/z^4_8/1

== system dt_toy_model_simulation/dt_SLS_gain1/z*Phi_x(z)-I/1//z^5 ==
  v : Inport
  1/z^5_{1..18} (18 alike) : DiscreteTransferFcn  Denominator=[1 0 0 0 0 0]
  Demux1 : Demux  Outputs=18
  Mux1 : Mux  Inputs=18
  Out1 : Outport
  wires:
  Demux1/8 -> 1/z^5_8/1
  1/z^5_8/1 -> Mux1/8
  Demux1/4 -> 1/z^5_4/1
  1/z^5_5/1 -> Mux1/5
  1/z^5_18/1 -> Mux1/18
  1/z^5_17/1 -> Mux1/17
  Demux1/5 -> 1/z^5_5/1
  Demux1/17 -> 1/z^5_17/1
  Demux1/14 -> 1/z^5_14/1
  1/z^5_16/1 -> Mux1/16
  1/z^5_14/1 -> Mux1/14
  Demux1/11 -> 1/z^5_11/1
  1/z^5_11/1 -> Mux1/11
  Demux1/16 -> 1/z^5_16/1
  1/z^5_4/1 -> Mux1/4
  1/z^5_10/1 -> Mux1/10
  Demux1/18 -> 1/z^5_18/1
  Demux1/13 -> 1/z^5_13/1
  1/z^5_13/1 -> Mux1/13
  1/z^5_12/1 -> Mux1/12
  Demux1/12 -> 1/z^5_12/1
  Demux1/15 -> 1/z^5_15/1
  1/z^5_15/1 -> Mux1/15
  Mux1/1 -> Out1/1
  1/z^5_6/1 -> Mux1/6
  1/z^5_2/1 -> Mux1/2
  Demux1/2 -> 1/z^5_2/1
  Demux1/6 -> 1/z^5_6/1
  v/1 -> Demux1/1
  1/z^5_1/1 -> Mux1/1
  Demux1/10 -> 1/z^5_10/1
  Demux1/1 -> 1/z^5_1/1
  1/z^5_3/1 -> Mux1/3
  1/z^5_7/1 -> Mux1/7
  Demux1/7 -> 1/z^5_7/1
  Demux1/9 -> 1/z^5_9/1
  1/z^5_9/1 -> Mux1/9
  Demux1/3 -> 1/z^5_3/1

== system dt_toy_model_simulation/dt_SLS_gain1/z*Phi_x(z)-I/1//z^6 ==
  v : Inport
  1/z^5_{1..18} (18 alike) : DiscreteTransferFcn  Denominator=[1 0 0 0 0 0 0]
  Demux1 : Demux  Outputs=18
  Mux1 : Mux  Inputs=18
  Out1 : Outport
  wires:
  Demux1/3 -> 1/z^5_3/1
  1/z^5_9/1 -> Mux1/9
  Demux1/9 -> 1/z^5_9/1
  Demux1/7 -> 1/z^5_7/1
  1/z^5_7/1 -> Mux1/7
  1/z^5_3/1 -> Mux1/3
  Demux1/1 -> 1/z^5_1/1
  Demux1/10 -> 1/z^5_10/1
  1/z^5_1/1 -> Mux1/1
  v/1 -> Demux1/1
  Demux1/6 -> 1/z^5_6/1
  Demux1/2 -> 1/z^5_2/1
  1/z^5_2/1 -> Mux1/2
  1/z^5_6/1 -> Mux1/6
  Mux1/1 -> Out1/1
  1/z^5_15/1 -> Mux1/15
  Demux1/15 -> 1/z^5_15/1
  Demux1/12 -> 1/z^5_12/1
  1/z^5_12/1 -> Mux1/12
  1/z^5_13/1 -> Mux1/13
  Demux1/13 -> 1/z^5_13/1
  Demux1/18 -> 1/z^5_18/1
  1/z^5_10/1 -> Mux1/10
  1/z^5_4/1 -> Mux1/4
  Demux1/16 -> 1/z^5_16/1
  1/z^5_11/1 -> Mux1/11
  Demux1/11 -> 1/z^5_11/1
  1/z^5_14/1 -> Mux1/14
  1/z^5_16/1 -> Mux1/16
  Demux1/14 -> 1/z^5_14/1
  Demux1/17 -> 1/z^5_17/1
  Demux1/5 -> 1/z^5_5/1
  1/z^5_17/1 -> Mux1/17
  1/z^5_18/1 -> Mux1/18
  1/z^5_5/1 -> Mux1/5
  Demux1/4 -> 1/z^5_4/1
  1/z^5_8/1 -> Mux1/8
  Demux1/8 -> 1/z^5_8/1

== system dt_toy_model_simulation/dt_SLS_gain2/z*Phi_u(z)/1//z1 ==
  v : Inport
  Demux : Demux  Outputs=18
  Discrete Transfer Fcn{,1..17} (18 alike) : DiscreteTransferFcn  Denominator=[1 0]
  Mux : Mux  Inputs=18
  u : Outport
  wires:
  Discrete Transfer Fcn11/1 -> Mux/12
  Discrete Transfer Fcn10/1 -> Mux/11
  Discrete Transfer Fcn9/1 -> Mux/10
  Discrete Transfer Fcn8/1 -> Mux/9
  Discrete Transfer Fcn7/1 -> Mux/8
  Discrete Transfer Fcn6/1 -> Mux/7
  Discrete Transfer Fcn5/1 -> Mux/6
  Discrete Transfer Fcn4/1 -> Mux/5
  Discrete Transfer Fcn3/1 -> Mux/4
  Discrete Transfer Fcn14/1 -> Mux/13
  Discrete Transfer Fcn15/1 -> Mux/14
  Discrete Transfer Fcn16/1 -> Mux/15
  Discrete Transfer Fcn17/1 -> Mux/16
  Discrete Transfer Fcn12/1 -> Mux/17
  Discrete Transfer Fcn13/1 -> Mux/18
  Demux/18 -> Discrete Transfer Fcn13/1
  Demux/17 -> Discrete Transfer Fcn12/1
  Demux/16 -> Discrete Transfer Fcn17/1
  Demux/15 -> Discrete Transfer Fcn16/1
  Demux/14 -> Discrete Transfer Fcn15/1
  Demux/13 -> Discrete Transfer Fcn14/1
  Demux/12 -> Discrete Transfer Fcn11/1
  Demux/11 -> Discrete Transfer Fcn10/1
  Demux/10 -> Discrete Transfer Fcn9/1
  Demux/9 -> Discrete Transfer Fcn8/1
  Demux/8 -> Discrete Transfer Fcn7/1
  Demux/7 -> Discrete Transfer Fcn6/1
  Demux/6 -> Discrete Transfer Fcn5/1
  Demux/5 -> Discrete Transfer Fcn4/1
  Demux/4 -> Discrete Transfer Fcn3/1
  v/1 -> Demux/1
  Mux/1 -> u/1
  Demux/3 -> Discrete Transfer Fcn2/1
  Demux/2 -> Discrete Transfer Fcn1/1
  Discrete Transfer Fcn/1 -> Mux/1
  Discrete Transfer Fcn2/1 -> Mux/3
  Demux/1 -> Discrete Transfer Fcn/1
  Discrete Transfer Fcn1/1 -> Mux/2

== system dt_toy_model_simulation/dt_SLS_gain2/z*Phi_u(z)/1//z^2 ==
  v : Inport
  1/z^{1..18} (18 alike) : DiscreteTransferFcn  Denominator=[1 0 0]
  Demux1 : Demux  Outputs=18
  Mux1 : Mux  Inputs=18
  u : Outport
  wires:
  Demux1/15 -> 1/z^15/1
  Demux1/17 -> 1/z^17/1
  1/z^9/1 -> Mux1/9
  Demux1/18 -> 1/z^18/1
  Demux1/11 -> 1/z^11/1
  Demux1/3 -> 1/z^3/1
  1/z^4/1 -> Mux1/4
  1/z^8/1 -> Mux1/8
  1/z^12/1 -> Mux1/12
  1/z^3/1 -> Mux1/3
  Demux1/8 -> 1/z^8/1
  v/1 -> Demux1/1
  1/z^18/1 -> Mux1/18
  1/z^2/1 -> Mux1/2
  1/z^14/1 -> Mux1/14
  Demux1/4 -> 1/z^4/1
  Demux1/16 -> 1/z^16/1
  1/z^10/1 -> Mux1/10
  Demux1/9 -> 1/z^9/1
  Demux1/5 -> 1/z^5/1
  1/z^5/1 -> Mux1/5
  Demux1/12 -> 1/z^12/1
  1/z^7/1 -> Mux1/7
  1/z^15/1 -> Mux1/15
  1/z^11/1 -> Mux1/11
  Demux1/13 -> 1/z^13/1
  1/z^6/1 -> Mux1/6
  1/z^1/1 -> Mux1/1
  Demux1/1 -> 1/z^1/1
  Demux1/2 -> 1/z^2/1
  Mux1/1 -> u/1
  1/z^13/1 -> Mux1/13
  Demux1/6 -> 1/z^6/1
  Demux1/14 -> 1/z^14/1
  1/z^17/1 -> Mux1/17
  Demux1/10 -> 1/z^10/1
  1/z^16/1 -> Mux1/16
  Demux1/7 -> 1/z^7/1

== system dt_toy_model_simulation/dt_SLS_gain2/z*Phi_u(z)/1//z^3 ==
  v : Inport
  1/z^3_{1..18} (18 alike) : DiscreteTransferFcn  Denominator=[1 0 0 0]
  Demux1 : Demux  Outputs=18
  Mux1 : Mux  Inputs=18
  u : Outport
  wires:
  Demux1/3 -> 1/z^3_3/1
  1/z^3_9/1 -> Mux1/9
  Demux1/9 -> 1/z^3_9/1
  Demux1/7 -> 1/z^3_7/1
  1/z^3_7/1 -> Mux1/7
  1/z^3_3/1 -> Mux1/3
  Demux1/1 -> 1/z^3_1/1
  Demux1/10 -> 1/z^3_10/1
  1/z^3_1/1 -> Mux1/1
  v/1 -> Demux1/1
  Demux1/6 -> 1/z^3_6/1
  Demux1/2 -> 1/z^3_2/1
  1/z^3_2/1 -> Mux1/2
  1/z^3_6/1 -> Mux1/6
  Mux1/1 -> u/1
  1/z^3_15/1 -> Mux1/15
  Demux1/15 -> 1/z^3_15/1
  Demux1/12 -> 1/z^3_12/1
  1/z^3_12/1 -> Mux1/12
  1/z^3_13/1 -> Mux1/13
  Demux1/13 -> 1/z^3_13/1
  Demux1/18 -> 1/z^3_18/1
  1/z^3_10/1 -> Mux1/10
  1/z^3_4/1 -> Mux1/4
  Demux1/16 -> 1/z^3_16/1
  1/z^3_11/1 -> Mux1/11
  Demux1/11 -> 1/z^3_11/1
  1/z^3_14/1 -> Mux1/14
  1/z^3_16/1 -> Mux1/16
  Demux1/14 -> 1/z^3_14/1
  Demux1/17 -> 1/z^3_17/1
  Demux1/5 -> 1/z^3_5/1
  1/z^3_17/1 -> Mux1/17
  1/z^3_18/1 -> Mux1/18
  1/z^3_5/1 -> Mux1/5
  Demux1/4 -> 1/z^3_4/1
  1/z^3_8/1 -> Mux1/8
  Demux1/8 -> 1/z^3_8/1

== system dt_toy_model_simulation/dt_SLS_gain2/z*Phi_u(z)/1//z^4 ==
  v : Inport
  1/z^4_{1..18} (18 alike) : DiscreteTransferFcn  Denominator=[1 0 0 0 0]
  Demux1 : Demux  Outputs=18
  Mux1 : Mux  Inputs=18
  u : Outport
  wires:
  Demux1/8 -> 1/z^4_8/1
  1/z^4_8/1 -> Mux1/8
  Demux1/4 -> 1/z^4_4/1
  1/z^4_5/1 -> Mux1/5
  1/z^4_18/1 -> Mux1/18
  1/z^4_17/1 -> Mux1/17
  Demux1/5 -> 1/z^4_5/1
  Demux1/17 -> 1/z^4_17/1
  Demux1/14 -> 1/z^4_13/1
  1/z^4_15/1 -> Mux1/16
  1/z^4_13/1 -> Mux1/14
  Demux1/11 -> 1/z^4_11/1
  1/z^4_11/1 -> Mux1/11
  Demux1/16 -> 1/z^4_15/1
  1/z^4_4/1 -> Mux1/4
  1/z^4_10/1 -> Mux1/10
  Demux1/18 -> 1/z^4_18/1
  Demux1/13 -> 1/z^4_16/1
  1/z^4_16/1 -> Mux1/13
  1/z^4_12/1 -> Mux1/12
  Demux1/12 -> 1/z^4_12/1
  Demux1/15 -> 1/z^4_14/1
  1/z^4_14/1 -> Mux1/15
  Mux1/1 -> u/1
  1/z^4_6/1 -> Mux1/6
  1/z^4_2/1 -> Mux1/2
  Demux1/2 -> 1/z^4_2/1
  Demux1/6 -> 1/z^4_6/1
  v/1 -> Demux1/1
  1/z^4_1/1 -> Mux1/1
  Demux1/10 -> 1/z^4_10/1
  Demux1/1 -> 1/z^4_1/1
  1/z^4_3/1 -> Mux1/3
  1/z^4_7/1 -> Mux1/7
  Demux1/7 -> 1/z^4_7/1
  Demux1/9 -> 1/z^4_9/1
  1/z^4_9/1 -> Mux1/9
  Demux1/3 -> 1/z^4_3/1

== system dt_toy_model_simulation/dt_SLS_gain2/z*Phi_u(z)/1//z^5 ==
  v : Inport
  1/z^5_{1..18} (18 alike) : DiscreteTransferFcn  Denominator=[1 0 0 0 0 0]
  Demux1 : Demux  Outputs=18
  Mux1 : Mux  Inputs=18
  u : Outport
  wires:
  Demux1/3 -> 1/z^5_3/1
  1/z^5_9/1 -> Mux1/9
  Demux1/9 -> 1/z^5_9/1
  Demux1/7 -> 1/z^5_7/1
  1/z^5_7/1 -> Mux1/7
  1/z^5_3/1 -> Mux1/3
  Demux1/1 -> 1/z^5_1/1
  Demux1/10 -> 1/z^5_10/1
  1/z^5_1/1 -> Mux1/1
  v/1 -> Demux1/1
  Demux1/6 -> 1/z^5_6/1
  Demux1/2 -> 1/z^5_2/1
  1/z^5_2/1 -> Mux1/2
  1/z^5_6/1 -> Mux1/6
  Mux1/1 -> u/1
  1/z^5_15/1 -> Mux1/15
  Demux1/15 -> 1/z^5_15/1
  Demux1/12 -> 1/z^5_12/1
  1/z^5_12/1 -> Mux1/12
  1/z^5_13/1 -> Mux1/13
  Demux1/13 -> 1/z^5_13/1
  Demux1/18 -> 1/z^5_18/1
  1/z^5_10/1 -> Mux1/10
  1/z^5_4/1 -> Mux1/4
  Demux1/16 -> 1/z^5_16/1
  1/z^5_11/1 -> Mux1/11
  Demux1/11 -> 1/z^5_11/1
  1/z^5_14/1 -> Mux1/14
  1/z^5_16/1 -> Mux1/16
  Demux1/14 -> 1/z^5_14/1
  Demux1/17 -> 1/z^5_17/1
  Demux1/5 -> 1/z^5_5/1
  1/z^5_17/1 -> Mux1/17
  1/z^5_18/1 -> Mux1/18
  1/z^5_5/1 -> Mux1/5
  Demux1/4 -> 1/z^5_4/1
  1/z^5_8/1 -> Mux1/8
  Demux1/8 -> 1/z^5_8/1

== system dt_toy_model_simulation/dt_SLS_gain2/z*Phi_u(z)/1//z^6 ==
  v : Inport
  1/z^5_{1..18} (18 alike) : DiscreteTransferFcn  Denominator=[1 0 0 0 0 0 0]
  Demux1 : Demux  Outputs=18
  Mux1 : Mux  Inputs=18
  Out1 : Outport
  wires:
  Demux1/8 -> 1/z^5_8/1
  1/z^5_8/1 -> Mux1/8
  Demux1/4 -> 1/z^5_4/1
  1/z^5_5/1 -> Mux1/5
  1/z^5_18/1 -> Mux1/18
  1/z^5_17/1 -> Mux1/17
  Demux1/5 -> 1/z^5_5/1
  Demux1/17 -> 1/z^5_17/1
  Demux1/14 -> 1/z^5_14/1
  1/z^5_16/1 -> Mux1/16
  1/z^5_14/1 -> Mux1/14
  Demux1/11 -> 1/z^5_11/1
  1/z^5_11/1 -> Mux1/11
  Demux1/16 -> 1/z^5_16/1
  1/z^5_4/1 -> Mux1/4
  1/z^5_10/1 -> Mux1/10
  Demux1/18 -> 1/z^5_18/1
  Demux1/13 -> 1/z^5_13/1
  1/z^5_13/1 -> Mux1/13
  1/z^5_12/1 -> Mux1/12
  Demux1/12 -> 1/z^5_12/1
  Demux1/15 -> 1/z^5_15/1
  1/z^5_15/1 -> Mux1/15
  Mux1/1 -> Out1/1
  1/z^5_6/1 -> Mux1/6
  1/z^5_2/1 -> Mux1/2
  Demux1/2 -> 1/z^5_2/1
  Demux1/6 -> 1/z^5_6/1
  v/1 -> Demux1/1
  1/z^5_1/1 -> Mux1/1
  Demux1/10 -> 1/z^5_10/1
  Demux1/1 -> 1/z^5_1/1
  1/z^5_3/1 -> Mux1/3
  1/z^5_7/1 -> Mux1/7
  Demux1/7 -> 1/z^5_7/1
  Demux1/9 -> 1/z^5_9/1
  1/z^5_9/1 -> Mux1/9
  Demux1/3 -> 1/z^5_3/1

== system dt_toy_model_simulation/dt_SLS_gain2/z*Phi_x(z)-I/1//z ==
  v : Inport
  Demux : Demux  Outputs=18
  Discrete Transfer Fcn{,1..17} (18 alike) : DiscreteTransferFcn  Denominator=[1 0]
  Mux : Mux  Inputs=18
  Out1 : Outport
  wires:
  Discrete Transfer Fcn11/1 -> Mux/12
  Discrete Transfer Fcn10/1 -> Mux/11
  Discrete Transfer Fcn9/1 -> Mux/10
  Discrete Transfer Fcn8/1 -> Mux/9
  Discrete Transfer Fcn7/1 -> Mux/8
  Discrete Transfer Fcn6/1 -> Mux/7
  Discrete Transfer Fcn5/1 -> Mux/6
  Discrete Transfer Fcn4/1 -> Mux/5
  Discrete Transfer Fcn3/1 -> Mux/4
  Discrete Transfer Fcn14/1 -> Mux/13
  Discrete Transfer Fcn15/1 -> Mux/14
  Discrete Transfer Fcn16/1 -> Mux/15
  Discrete Transfer Fcn17/1 -> Mux/16
  Discrete Transfer Fcn12/1 -> Mux/17
  Discrete Transfer Fcn13/1 -> Mux/18
  Demux/18 -> Discrete Transfer Fcn13/1
  Demux/17 -> Discrete Transfer Fcn12/1
  Demux/16 -> Discrete Transfer Fcn17/1
  Demux/15 -> Discrete Transfer Fcn16/1
  Demux/14 -> Discrete Transfer Fcn15/1
  Demux/13 -> Discrete Transfer Fcn14/1
  Demux/12 -> Discrete Transfer Fcn11/1
  Demux/11 -> Discrete Transfer Fcn10/1
  Demux/10 -> Discrete Transfer Fcn9/1
  Demux/9 -> Discrete Transfer Fcn8/1
  Demux/8 -> Discrete Transfer Fcn7/1
  Demux/7 -> Discrete Transfer Fcn6/1
  Demux/6 -> Discrete Transfer Fcn5/1
  Demux/5 -> Discrete Transfer Fcn4/1
  Demux/4 -> Discrete Transfer Fcn3/1
  v/1 -> Demux/1
  Mux/1 -> Out1/1
  Demux/3 -> Discrete Transfer Fcn2/1
  Demux/2 -> Discrete Transfer Fcn1/1
  Discrete Transfer Fcn/1 -> Mux/1
  Discrete Transfer Fcn2/1 -> Mux/3
  Demux/1 -> Discrete Transfer Fcn/1
  Discrete Transfer Fcn1/1 -> Mux/2

== system dt_toy_model_simulation/dt_SLS_gain2/z*Phi_x(z)-I/1//z^2 ==
  v : Inport
  1/z^{1..18} (18 alike) : DiscreteTransferFcn  Denominator=[1 0 0]
  Demux1 : Demux  Outputs=18
  Mux1 : Mux  Inputs=18
  Out1 : Outport
  wires:
  Demux1/15 -> 1/z^15/1
  Demux1/17 -> 1/z^17/1
  1/z^9/1 -> Mux1/9
  Demux1/18 -> 1/z^18/1
  Demux1/11 -> 1/z^11/1
  Demux1/3 -> 1/z^3/1
  1/z^4/1 -> Mux1/4
  1/z^8/1 -> Mux1/8
  1/z^12/1 -> Mux1/12
  1/z^3/1 -> Mux1/3
  Demux1/8 -> 1/z^8/1
  v/1 -> Demux1/1
  1/z^18/1 -> Mux1/18
  1/z^2/1 -> Mux1/2
  1/z^14/1 -> Mux1/14
  Demux1/4 -> 1/z^4/1
  Demux1/16 -> 1/z^16/1
  1/z^10/1 -> Mux1/10
  Demux1/9 -> 1/z^9/1
  Demux1/5 -> 1/z^5/1
  1/z^5/1 -> Mux1/5
  Demux1/12 -> 1/z^12/1
  1/z^7/1 -> Mux1/7
  1/z^15/1 -> Mux1/15
  1/z^11/1 -> Mux1/11
  Demux1/13 -> 1/z^13/1
  1/z^6/1 -> Mux1/6
  1/z^1/1 -> Mux1/1
  Demux1/1 -> 1/z^1/1
  Demux1/2 -> 1/z^2/1
  Mux1/1 -> Out1/1
  1/z^13/1 -> Mux1/13
  Demux1/6 -> 1/z^6/1
  Demux1/14 -> 1/z^14/1
  1/z^17/1 -> Mux1/17
  Demux1/10 -> 1/z^10/1
  1/z^16/1 -> Mux1/16
  Demux1/7 -> 1/z^7/1

== system dt_toy_model_simulation/dt_SLS_gain2/z*Phi_x(z)-I/1//z^3 ==
  v : Inport
  1/z^3_{1..18} (18 alike) : DiscreteTransferFcn  Denominator=[1 0 0 0]
  Demux1 : Demux  Outputs=18
  Mux1 : Mux  Inputs=18
  Out1 : Outport
  wires:
  Demux1/3 -> 1/z^3_3/1
  1/z^3_9/1 -> Mux1/9
  Demux1/9 -> 1/z^3_9/1
  Demux1/7 -> 1/z^3_7/1
  1/z^3_7/1 -> Mux1/7
  1/z^3_3/1 -> Mux1/3
  Demux1/1 -> 1/z^3_1/1
  Demux1/10 -> 1/z^3_10/1
  1/z^3_1/1 -> Mux1/1
  v/1 -> Demux1/1
  Demux1/6 -> 1/z^3_6/1
  Demux1/2 -> 1/z^3_2/1
  1/z^3_2/1 -> Mux1/2
  1/z^3_6/1 -> Mux1/6
  Mux1/1 -> Out1/1
  1/z^3_15/1 -> Mux1/15
  Demux1/15 -> 1/z^3_15/1
  Demux1/12 -> 1/z^3_12/1
  1/z^3_12/1 -> Mux1/12
  1/z^3_13/1 -> Mux1/13
  Demux1/13 -> 1/z^3_13/1
  Demux1/18 -> 1/z^3_18/1
  1/z^3_10/1 -> Mux1/10
  1/z^3_4/1 -> Mux1/4
  Demux1/16 -> 1/z^3_16/1
  1/z^3_11/1 -> Mux1/11
  Demux1/11 -> 1/z^3_11/1
  1/z^3_14/1 -> Mux1/14
  1/z^3_16/1 -> Mux1/16
  Demux1/14 -> 1/z^3_14/1
  Demux1/17 -> 1/z^3_17/1
  Demux1/5 -> 1/z^3_5/1
  1/z^3_17/1 -> Mux1/17
  1/z^3_18/1 -> Mux1/18
  1/z^3_5/1 -> Mux1/5
  Demux1/4 -> 1/z^3_4/1
  1/z^3_8/1 -> Mux1/8
  Demux1/8 -> 1/z^3_8/1

== system dt_toy_model_simulation/dt_SLS_gain2/z*Phi_x(z)-I/1//z^4 ==
  v : Inport
  1/z^4_{1..18} (18 alike) : DiscreteTransferFcn  Denominator=[1 0 0 0 0]
  Demux1 : Demux  Outputs=18
  Mux1 : Mux  Inputs=18
  Out1 : Outport
  wires:
  Demux1/8 -> 1/z^4_8/1
  1/z^4_8/1 -> Mux1/8
  Demux1/4 -> 1/z^4_4/1
  1/z^4_5/1 -> Mux1/5
  1/z^4_18/1 -> Mux1/18
  1/z^4_17/1 -> Mux1/17
  Demux1/5 -> 1/z^4_5/1
  Demux1/17 -> 1/z^4_17/1
  Demux1/14 -> 1/z^4_13/1
  1/z^4_15/1 -> Mux1/16
  1/z^4_13/1 -> Mux1/14
  Demux1/11 -> 1/z^4_11/1
  1/z^4_11/1 -> Mux1/11
  Demux1/16 -> 1/z^4_15/1
  1/z^4_4/1 -> Mux1/4
  1/z^4_10/1 -> Mux1/10
  Demux1/18 -> 1/z^4_18/1
  Demux1/13 -> 1/z^4_16/1
  1/z^4_16/1 -> Mux1/13
  1/z^4_12/1 -> Mux1/12
  Demux1/12 -> 1/z^4_12/1
  Demux1/15 -> 1/z^4_14/1
  1/z^4_14/1 -> Mux1/15
  Mux1/1 -> Out1/1
  1/z^4_6/1 -> Mux1/6
  1/z^4_2/1 -> Mux1/2
  Demux1/2 -> 1/z^4_2/1
  Demux1/6 -> 1/z^4_6/1
  v/1 -> Demux1/1
  1/z^4_1/1 -> Mux1/1
  Demux1/10 -> 1/z^4_10/1
  Demux1/1 -> 1/z^4_1/1
  1/z^4_3/1 -> Mux1/3
  1/z^4_7/1 -> Mux1/7
  Demux1/7 -> 1/z^4_7/1
  Demux1/9 -> 1/z^4_9/1
  1/z^4_9/1 -> Mux1/9
  Demux1/3 -> 1/z^4_3/1

== system dt_toy_model_simulation/dt_SLS_gain2/z*Phi_x(z)-I/1//z^5 ==
  v : Inport
  1/z^5_{1..18} (18 alike) : DiscreteTransferFcn  Denominator=[1 0 0 0 0 0]
  Demux1 : Demux  Outputs=18
  Mux1 : Mux  Inputs=18
  Out1 : Outport
  wires:
  Demux1/3 -> 1/z^5_3/1
  1/z^5_9/1 -> Mux1/9
  Demux1/9 -> 1/z^5_9/1
  Demux1/7 -> 1/z^5_7/1
  1/z^5_7/1 -> Mux1/7
  1/z^5_3/1 -> Mux1/3
  Demux1/1 -> 1/z^5_1/1
  Demux1/10 -> 1/z^5_10/1
  1/z^5_1/1 -> Mux1/1
  v/1 -> Demux1/1
  Demux1/6 -> 1/z^5_6/1
  Demux1/2 -> 1/z^5_2/1
  1/z^5_2/1 -> Mux1/2
  1/z^5_6/1 -> Mux1/6
  Mux1/1 -> Out1/1
  1/z^5_15/1 -> Mux1/15
  Demux1/15 -> 1/z^5_15/1
  Demux1/12 -> 1/z^5_12/1
  1/z^5_12/1 -> Mux1/12
  1/z^5_13/1 -> Mux1/13
  Demux1/13 -> 1/z^5_13/1
  Demux1/18 -> 1/z^5_18/1
  1/z^5_10/1 -> Mux1/10
  1/z^5_4/1 -> Mux1/4
  Demux1/16 -> 1/z^5_16/1
  1/z^5_11/1 -> Mux1/11
  Demux1/11 -> 1/z^5_11/1
  1/z^5_14/1 -> Mux1/14
  1/z^5_16/1 -> Mux1/16
  Demux1/14 -> 1/z^5_14/1
  Demux1/17 -> 1/z^5_17/1
  Demux1/5 -> 1/z^5_5/1
  1/z^5_17/1 -> Mux1/17
  1/z^5_18/1 -> Mux1/18
  1/z^5_5/1 -> Mux1/5
  Demux1/4 -> 1/z^5_4/1
  1/z^5_8/1 -> Mux1/8
  Demux1/8 -> 1/z^5_8/1

== system dt_toy_model_simulation/dt_SLS_gain2/z*Phi_x(z)-I/1//z^6 ==
  v : Inport
  1/z^5_{1..18} (18 alike) : DiscreteTransferFcn  Denominator=[1 0 0 0 0 0 0]
  Demux1 : Demux  Outputs=18
  Mux1 : Mux  Inputs=18
  Out1 : Outport
  wires:
  Demux1/8 -> 1/z^5_8/1
  1/z^5_8/1 -> Mux1/8
  Demux1/4 -> 1/z^5_4/1
  1/z^5_5/1 -> Mux1/5
  1/z^5_18/1 -> Mux1/18
  1/z^5_17/1 -> Mux1/17
  Demux1/5 -> 1/z^5_5/1
  Demux1/17 -> 1/z^5_17/1
  Demux1/14 -> 1/z^5_14/1
  1/z^5_16/1 -> Mux1/16
  1/z^5_14/1 -> Mux1/14
  Demux1/11 -> 1/z^5_11/1
  1/z^5_11/1 -> Mux1/11
  Demux1/16 -> 1/z^5_16/1
  1/z^5_4/1 -> Mux1/4
  1/z^5_10/1 -> Mux1/10
  Demux1/18 -> 1/z^5_18/1
  Demux1/13 -> 1/z^5_13/1
  1/z^5_13/1 -> Mux1/13
  1/z^5_12/1 -> Mux1/12
  Demux1/12 -> 1/z^5_12/1
  Demux1/15 -> 1/z^5_15/1
  1/z^5_15/1 -> Mux1/15
  Mux1/1 -> Out1/1
  1/z^5_6/1 -> Mux1/6
  1/z^5_2/1 -> Mux1/2
  Demux1/2 -> 1/z^5_2/1
  Demux1/6 -> 1/z^5_6/1
  v/1 -> Demux1/1
  1/z^5_1/1 -> Mux1/1
  Demux1/10 -> 1/z^5_10/1
  Demux1/1 -> 1/z^5_1/1
  1/z^5_3/1 -> Mux1/3
  1/z^5_7/1 -> Mux1/7
  Demux1/7 -> 1/z^5_7/1
  Demux1/9 -> 1/z^5_9/1
  1/z^5_9/1 -> Mux1/9
  Demux1/3 -> 1/z^5_3/1

== matlab function dt_toy_model_simulation/dt_SLS_gain1/z*Phi_u(z)/MATLAB Function5 ==
  data: u input; Mat input; y output
function y = leftMult(u,Mat)

y = real(Mat)*u;

== matlab function dt_toy_model_simulation/dt_SLS_gain1/z*Phi_u(z)/MATLAB Function6 ==
  data: u input; Mat input; y output
function y = leftMult(u,Mat)

y = real(Mat)*u;

== matlab function dt_toy_model_simulation/dt_SLS_gain1/z*Phi_u(z)/MATLAB Function ==
  data: u input; Mat input; y output
function y = leftMult(u,Mat)

y = real(Mat)*u;

== matlab function dt_toy_model_simulation/dt_SLS_gain1/z*Phi_x(z)-I/MATLAB Function ==
  data: u input; Mat input; y output
function y = leftMult(u,Mat)

y = Mat*u;

== matlab function dt_toy_model_simulation/dt_SLS_gain1/z*Phi_x(z)-I/MATLAB Function1 ==
  data: u input; Mat input; y output
function y = leftMult(u,Mat)

y = Mat*u;

== matlab function dt_toy_model_simulation/dt_SLS_gain2/z*Phi_u(z)/MATLAB Function6 ==
  data: u input; Mat input; y output
function y = leftMult(u,Mat)

y = real(Mat)*u;

== matlab function dt_toy_model_simulation/dt_SLS_gain1/z*Phi_x(z)-I/MATLAB Function2 ==
  data: u input; Mat input; y output
function y = leftMult(u,Mat)

y = Mat*u;

== matlab function dt_toy_model_simulation/dt_SLS_gain1/z*Phi_x(z)-I/MATLAB Function3 ==
  data: u input; Mat input; y output
function y = leftMult(u,Mat)

y = Mat*u;

== matlab function dt_toy_model_simulation/dt_SLS_gain1/z*Phi_x(z)-I/MATLAB Function4 ==
  data: u input; Mat input; y output
function y = leftMult(u,Mat)

y = Mat*u;

== matlab function dt_toy_model_simulation/dt_SLS_gain1/z*Phi_x(z)-I/MATLAB Function5 ==
  data: u input; Mat input; y output
function y = leftMult(u,Mat)

y = Mat*u;

== matlab function dt_toy_model_simulation/OpenLoopModel ==
  data: Ac input; Bc input; x input; u input; dx output
function dx = ct_ss_model(Ac,Bc,x,u)

dx = Ac*x+Bc*u;

== matlab function dt_toy_model_simulation/dt_SLS_gain2/z*Phi_u(z)/MATLAB Function2 ==
  data: u input; Mat input; y output
function y = leftMult(u,Mat)

y = real(Mat)*u;

== matlab function dt_toy_model_simulation/dt_SLS_gain1/z*Phi_u(z)/MATLAB Function1 ==
  data: u input; Mat input; y output
function y = leftMult(u,Mat)

y = real(Mat)*u;

== matlab function dt_toy_model_simulation/dt_SLS_gain2/z*Phi_u(z)/MATLAB Function3 ==
  data: u input; Mat input; y output
function y = leftMult(u,Mat)

y = real(Mat)*u;

== matlab function dt_toy_model_simulation/dt_SLS_gain2/z*Phi_u(z)/MATLAB Function4 ==
  data: u input; Mat input; y output
function y = leftMult(u,Mat)

y = real(Mat)*u;

== matlab function dt_toy_model_simulation/dt_SLS_gain2/z*Phi_u(z)/MATLAB Function5 ==
  data: u input; Mat input; y output
function y = leftMult(u,Mat)

y = real(Mat)*u;

== matlab function dt_toy_model_simulation/dt_SLS_gain2/z*Phi_x(z)-I/MATLAB Function ==
  data: u input; Mat input; y output
function y = leftMult(u,Mat)

y = Mat*u;

== matlab function dt_toy_model_simulation/dt_SLS_gain2/z*Phi_x(z)-I/MATLAB Function1 ==
  data: u input; Mat input; y output
function y = leftMult(u,Mat)

y = Mat*u;

== matlab function dt_toy_model_simulation/dt_SLS_gain2/z*Phi_x(z)-I/MATLAB Function2 ==
  data: u input; Mat input; y output
function y = leftMult(u,Mat)

y = Mat*u;

== matlab function dt_toy_model_simulation/dt_SLS_gain2/z*Phi_x(z)-I/MATLAB Function4 ==
  data: u input; Mat input; y output
function y = leftMult(u,Mat)

y = Mat*u;

== matlab function dt_toy_model_simulation/dt_SLS_gain2/z*Phi_x(z)-I/MATLAB Function5 ==
  data: u input; Mat input; y output
function y = leftMult(u,Mat)

y = Mat*u;

== matlab function dt_toy_model_simulation/OpenLoopModel2 ==
  data: x input; u input; delta_x output
function delta_x = scalar_model(x,u)
Ad = 2;
Bd = 1;

delta_x = Ad*x+Bd*u;

== matlab function dt_toy_model_simulation/MATLAB Function3 ==
  data: in input; Mat input; out output
function out = leftMult(in,Mat)

out = real(Mat)*in;

== matlab function dt_toy_model_simulation/dt_SLS_gain1/z*Phi_u(z)/MATLAB Function2 ==
  data: u input; Mat input; y output
function y = leftMult(u,Mat)

y = real(Mat)*u;

== matlab function dt_toy_model_simulation/dt_SLS_gain1/z*Phi_u(z)/MATLAB Function3 ==
  data: u input; Mat input; y output
function y = leftMult(u,Mat)

y = real(Mat)*u;

== matlab function dt_toy_model_simulation/dt_SLS_gain2/z*Phi_u(z)/MATLAB Function ==
  data: u input; Mat input; y output
function y = leftMult(u,Mat)

y = real(Mat)*u;

== matlab function dt_toy_model_simulation/dt_SLS_gain2/z*Phi_u(z)/MATLAB Function1 ==
  data: u input; Mat input; y output
function y = leftMult(u,Mat)

y = real(Mat)*u;

== matlab function dt_toy_model_simulation/dt_SLS_gain1/z*Phi_u(z)/MATLAB Function4 ==
  data: u input; Mat input; y output
function y = leftMult(u,Mat)

y = real(Mat)*u;
